simulink model "pid_design"  (R2016a)
settings: Solver=ode4  StartTime=0.0  StopTime=10.0  RelTol=1e-3
settings Model: Creator=henri  LastModifiedBy=henri
settings OptimizationCC: BlockReduction=off  DefaultParameterBehavior=Inlined  BufferReuse=off

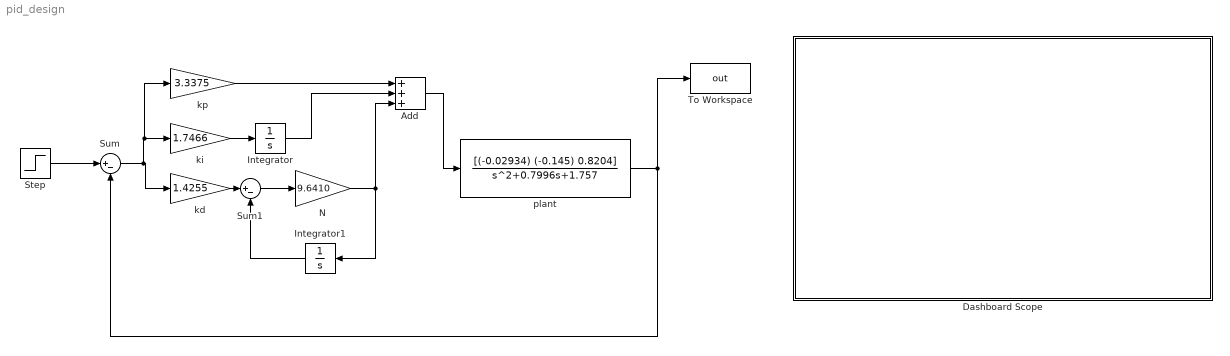
== system pid_design ==
  Add : Sum  Inputs=+++
  Dashboard Scope : Subsystem  DialogController=hmiCreateDDGDialog  IsWebBlock=on  mask(MWDashboardBlock){webBlockId=e872fcda-b87c-47a2-a194-b20f90f8cab5, webBlockType=sdiscope, ShowInitialText=on, HMISrcModelName=pid_design}
      mask prompts: webBlockId "WebBlock Id"; webBlockType "WebBlock Type"; HMISrcModelName "Source Model"
      mask Help: helpview([docroot '/mapfiles/simulink.map'], 'hmi_scope')
      mask Display:
      | if strcmp(get_param(bdroot(gcb),'BlockDiagramType'), 'library')
      |     image([(matlabroot) '/toolbox/simulink/hmi/icons/DashboardScope.png']);
      | end
  Integrator : Integrator
  Integrator1 : Integrator
  N : Gain  Gain=9.6410
  Step : Step  Time=0.5  After=0.9  SampleTime=0  VectorParams1D=off  ZeroCross=off
  Sum : Sum  Inputs=|+-
  Sum1 : Sum  Inputs=|+-
  To Workspace : ToWorkspace  VariableName=out  SaveFormat=Timeseries  SampleTime=-1
  kd : Gain  Gain=1.4255
  ki : Gain  Gain=1.7466
  kp : Gain  Gain=3.3375
  plant : TransferFcn  Numerator=[(-0.02934) (-0.145) 0.8204]  Denominator=[1 0.7996 1.757]
  wires:
  kp/1 -> Add/1
  ki/1 -> Integrator/1
  plant/1 -> Sum/2, To Workspace/1
  Integrator/1 -> Add/2
  Step/1 -> Sum/1
  Add/1 -> plant/1
  Sum/1 -> kp/1, ki/1, kd/1
  kd/1 -> Sum1/1
  Sum1/1 -> N/1
  N/1 -> Add/3, Integrator1/1
  Integrator1/1 -> Sum1/2

== system pid_design/Dashboard Scope ==
